simulink model "LongControl"  (R2018b)
settings: Solver=FixedStepAuto  StartTime=0.0  StopTime=100  FixedStep=0.1  RelTol=1e-3
values from neighbouring files (symbols this model uses):
  A = 1.5    [longparams.m]    (also in makeparams.m = [-(2*Cf+2*Cr)/m/Vx, 0, -Vx-(2*Cf*lf-2*Cr*lr)/m/Vx, 0)
  Cd = 0.3    [longparams.m]
  g = 9.8    [longparams.m]
  id = 7.91    [longparams.m]
  ig = 1.9370    (= 1.937)    [longparams.m]
  m = 296    [longparams.m]    (also in makeparams.m = 1575)
  mt = m + Jw/(Rw^2)    (= 473.514792899)    [longparams.m]
  Rho = 1.29    [longparams.m]
  Rw = 0.26    [longparams.m]
  Theta = 0    [longparams.m]
undefined symbols (not defined in the file or in its folder): magnitude
libraries: autolibshared x1, simulink x1
settings Model: Creator=reiserbalazs  LastModifiedBy=reiserbalazs

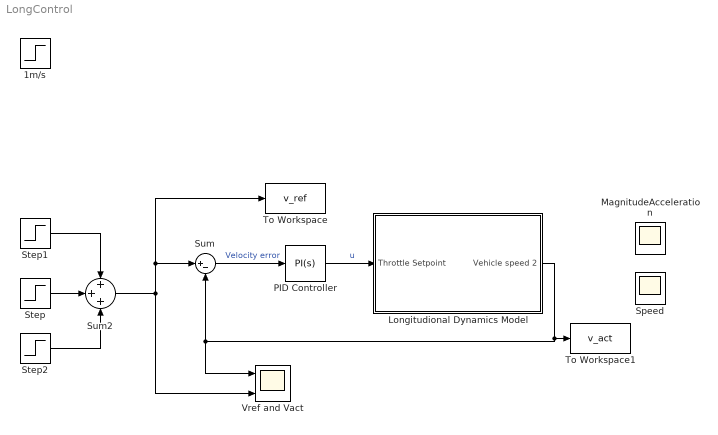
== system LongControl ==
  1m/s : Step  SampleTime=0
  Longitudional Dynamics Model : Subsystem
  MagnitudeAcceleration : Scope
  PID Controller : simulink/Continuous/PID Controller  Controller=PI  Form=Parallel  TimeDomain=Continuous-time  SampleTime=-1  IntegratorMethod=Forward Euler  FilterMethod=Forward Euler  ControllerParametersSource=internal  P=40  I=1.75  D=0  UseFilter=on  N=100  TunerSelectOption=Transfer Function Based (PID Tuner App)  InitialConditionSource=internal  InitialConditionForIntegrator=0  InitialConditionForFilter=0  DifferentiatorICPrevScaledInput=0  ExternalReset=none  TrackingMode=off  Kt=1  LimitOutput=on  UpperSaturationLimit=inf  LowerSaturationLimit=-inf  LinearizeAsGain=on  AntiWindupMode=clamping  Kb=1  POutMin=[]  POutMax=[]  IOutMin=[]  IOutMax=[]  DOutMin=[]  DOutMax=[]  NOutMin=[]  NOutMax=[]  SumOutMin=[]  SumOutMax=[]  SaturationOutMin=[]  SaturationOutMax=[]  PParamMin=[]  PParamMax=[]  IParamMin=[]  IParamMax=[]  DParamMin=[]  DParamMax=[]  NParamMin=[]  NParamMax=[]  KbParamMin=[]  KbParamMax=[]  KtParamMin=[]  KtParamMax=[]  KbOutMin=[]  KbOutMax=[]  KtOutMin=[]  KtOutMax=[]  IntegratorOutMin=[]  IntegratorOutMax=[]  FilterOutMin=[]  FilterOutMax=[]  SumI1OutMin=[]  SumI1OutMax=[]  SumI2OutMin=[]  SumI2OutMax=[]  SumI3OutMin=[]  SumI3OutMax=[]  SumI4OutMin=[]  SumI4OutMax=[]  SumDOutMin=[]  SumDOutMax=[]  DifferentiatorOutMin=[]  DifferentiatorOutMax=[]  FilterDiffOutCoefMin=[]  FilterDiffOutCoefMax=[]  ReciprocalOutMin=[]  ReciprocalOutMax=[]  SumDenOutMin=[]  SumDenOutMax=[]  SumNumOutMin=[]  SumNumOutMax=[]  DivideOutMin=[]  DivideOutMax=[]  IntegratorContinuousStateAttributes=''  IntegratorStateMustResolveToSignalObject=off  IntegratorRTWStateStorageClass=Auto  FilterContinuousStateAttributes=''  FilterStateMustResolveToSignalObject=off  FilterRTWStateStorageClass=Auto  ParallelPVariant=InternalParameters  IdealPVariant=Disabled  IVariant=InternalParameters  DVariant=Disabled  IntegratorVariant=Continuous  SatVariant=Enabled  AWVariant=ContClampingParallel  PCopyVariant=Disabled  TRVariant=Disabled  FdbkBlocksVariant=Forward  IdealPFdbkVariant=Disabled  SatFdbkVariant=Disabled  DerivativeFilterVariant=Disabled  NVariant=Disabled  NCopyVariant=Disabled_SignalSpec  FilterICVariant=Disabled  IntegratorICVariant=InternalICs  ExternalResetVariant=Disabled  TRSumVariant=Passthrough  SumFdbkVariant=Disabled  SumVariant=Sum_PI
  Speed : Scope
  Step : Step  Time=0  After=10  SampleTime=0
  Step1 : Step  Time=30  After=20  SampleTime=0
  Step2 : Step  Time=60  After=-10  SampleTime=0
  Sum : Sum  Inputs=|+-
  Sum2 : Sum  Inputs=+++
  To Workspace : ToWorkspace  VariableName=v_ref  SaveFormat=Timeseries  SampleTime=-1
  To Workspace1 : ToWorkspace  VariableName=v_act  SaveFormat=Timeseries  SampleTime=-1
  Vref and Vact : Scope  NumInputPorts=2
  wires:
  PID Controller/1 -> Longitudional Dynamics Model/1(Throttle Setpoint)  "u"
  Sum/1 -> PID Controller/1  "Velocity error"
  Step/1 -> Sum2/2
  Step1/1 -> Sum2/1
  Longitudional Dynamics Model/1(Vehicle speed 2) -> To Workspace1/1, Sum/2, Vref and Vact/1
  Step2/1 -> Sum2/3
  Sum2/1 -> To Workspace/1, Sum/1, Vref and Vact/2

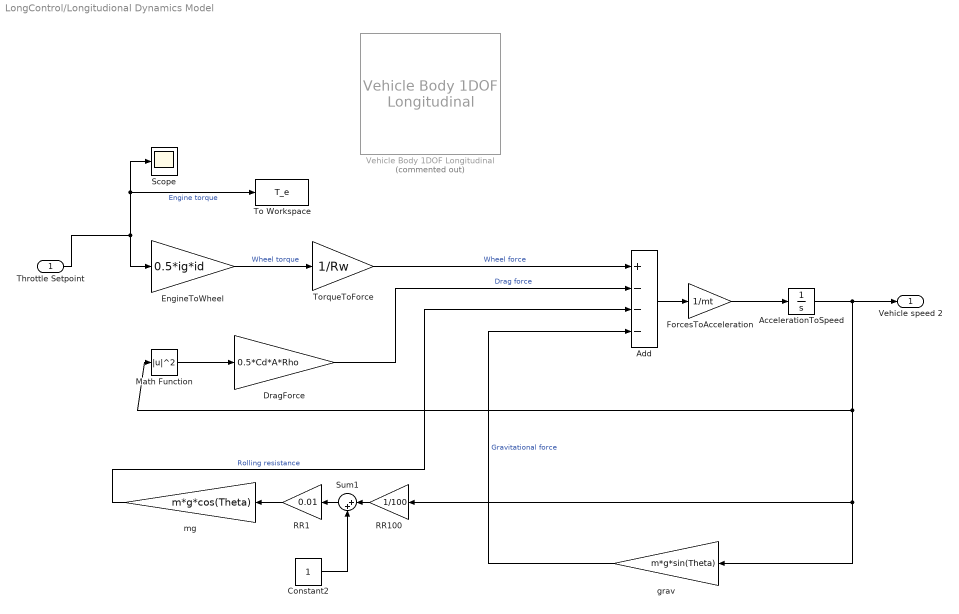
== system LongControl/Longitudional Dynamics Model ==
  Throttle Setpoint : Inport
  AccelerationToSpeed : Integrator
  Add : Sum  Inputs=+---
  Constant2 : Constant
  DragForce : Gain  Gain=0.5*Cd*A*Rho
  EngineToWheel : Gain  Gain=0.5*ig*id
  ForcesToAcceleration : Gain  Gain=1/mt
  Math Function : Math  Operator=magnitude^2  SaturateOnIntegerOverflow=on
  RR1 : Gain  Gain=0.01
  RR100 : Gain  Gain=1/100
  Scope : Scope
  Sum1 : Sum  Inputs=|++
  To Workspace : ToWorkspace  VariableName=T_e  SaveFormat=Timeseries  SampleTime=-1
  TorqueToForce : Gain  Gain=1/Rw
  Vehicle Body 1DOF Longitudinal : autolibshared/Vehicle Body 1DOF Longitudinal  Commented=on  VariantControl=SL  aMode=1  NF=2  NR=2  m=300  a=1.1  b=0.9  h=.2  Cd=.3  Af=2.1  x_o=0  xdot_o=0  Pabs=101325  T=273  g=9.81
      settings: SourceProductName=Powertrain Blockset  SourceProductBaseCode=PW
  grav : Gain  Gain=m*g*sin(Theta)
  mg : Gain  Gain=m*g*cos(Theta)
  Vehicle speed 2 : Outport
  wires:
  Add/1 -> ForcesToAcceleration/1
  DragForce/1 -> Add/2  "Drag force"
  AccelerationToSpeed/1 -> grav/1, RR100/1, Math Function/1, Vehicle speed 2/1
  ForcesToAcceleration/1 -> AccelerationToSpeed/1
  Math Function/1 -> DragForce/1
  TorqueToForce/1 -> Add/1  "Wheel force"
  EngineToWheel/1 -> TorqueToForce/1  "Wheel torque"
  RR100/1 -> Sum1/1
  Constant2/1 -> Sum1/2
  Sum1/1 -> RR1/1
  RR1/1 -> mg/1
  mg/1 -> Add/3  "Rolling resistance"
  grav/1 -> Add/4  "Gravitational force"
  Throttle Setpoint/1 -> EngineToWheel/1, To Workspace/1, Scope/1  "Engine torque"
